simulink model "omav_allocation"  (R2020a)
settings: Solver=VariableStepAuto  StartTime=0.0  StopTime=50  RelTol=1e-3
undefined symbols (not defined in the file): params
libraries: simulink x12
settings Model: Creator=daniel  LastModifiedBy=daniel

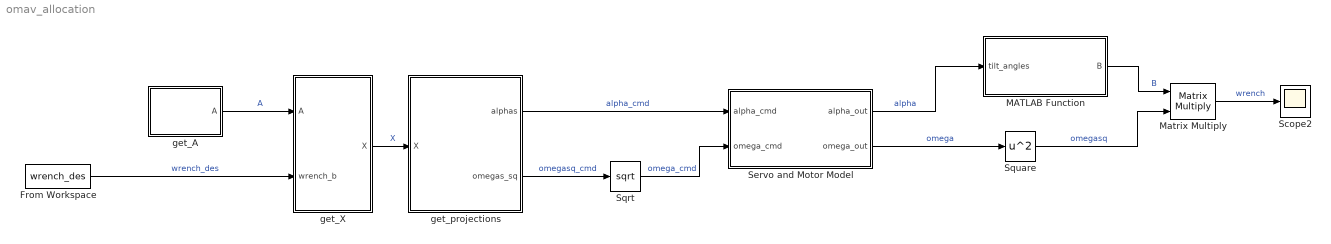
== system omav_allocation ==
  " get_A" : MATLAB Function  TreatAsAtomicUnit=on
  From Workspace : FromWorkspace  VariableName=wrench_des  SampleTime=params.sampling_time
  MATLAB Function : MATLAB Function  TreatAsAtomicUnit=on
  Matrix Multiply : Product  Multiplication=Matrix(*)
  Scope2 : Scope
  Servo and Motor Model : Subsystem
  Sqrt : Sqrt  SaturateOnIntegerOverflow=on
  Square : Math  Operator=square  SaturateOnIntegerOverflow=on
  get_X : MATLAB Function  TreatAsAtomicUnit=on
  get_projections : MATLAB Function  TreatAsAtomicUnit=on
  wires:
  From Workspace/1 -> get_X/2(wrench_b)  "wrench_des"
  " get_A"/1(A) -> get_X/1(A)  "A"
  get_X/1(X) -> get_projections/1(X)  "X"
  get_projections/1(alphas) -> Servo and Motor Model/1(alpha_cmd)  "alpha_cmd"
  MATLAB Function/1(B) -> Matrix Multiply/1  "B"
  get_projections/2(omegas_sq) -> Sqrt/1  "omegasq_cmd"
  Matrix Multiply/1 -> Scope2/1  "wrench"
  Sqrt/1 -> Servo and Motor Model/2(omega_cmd)  "omega_cmd"
  Servo and Motor Model/1(alpha_out) -> MATLAB Function/1(tilt_angles)  "alpha"
  Servo and Motor Model/2(omega_out) -> Square/1  "omega"
  Square/1 -> Matrix Multiply/2  "omegasq"

== system omav_allocation/Servo and Motor Model ==
  alpha_cmd : Inport
  omega_cmd : Inport  Port=2
  all_rotors_subsystem1 : Subsystem
      mask Display: image('images/brushless.JPG'); % Use "Edit Image" on toolstrip to change.
  all_servos_subsystem1 : Subsystem
      mask Display: image('images/servo.jpg'); % Use "Edit Image" on toolstrip to change.
  alpha_out : Outport
  omega_out : Outport  Port=2
  wires:
  alpha_cmd/1 -> all_servos_subsystem1/1(alphas_cmd)  "alpha_cmd"
  all_rotors_subsystem1/1(omegas_out) -> omega_out/1  "omega_out"
  all_servos_subsystem1/1(alphas_out) -> alpha_out/1  "alpha_out"
  omega_cmd/1 -> all_rotors_subsystem1/1(omegas_cmd)  "omega_cmd"

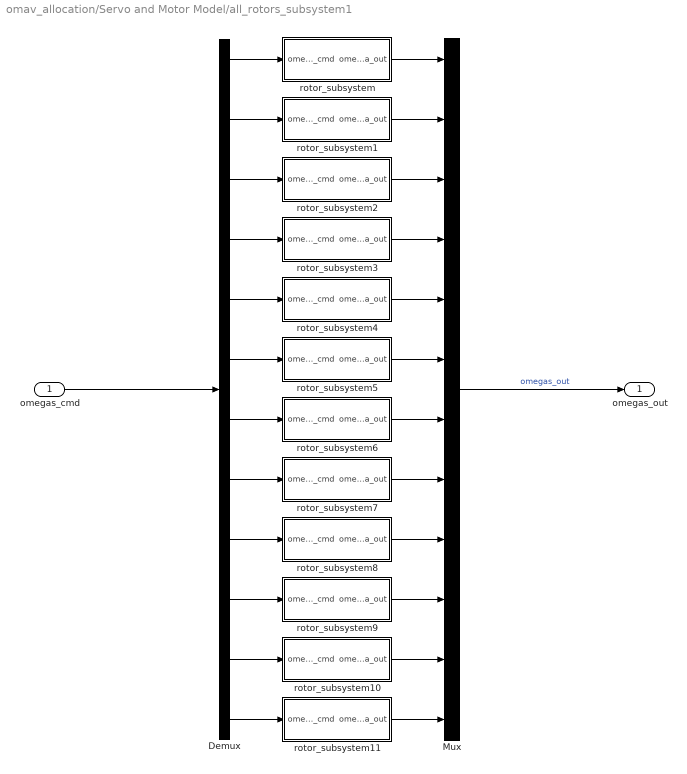
== system omav_allocation/Servo and Motor Model/all_rotors_subsystem1 ==
  omegas_cmd : Inport
  Demux : Demux  Outputs=12
  Mux : Mux  Inputs=12
  rotor_subsystem : Subsystem
  rotor_subsystem1 : Subsystem
  rotor_subsystem10 : Subsystem
  rotor_subsystem11 : Subsystem
  rotor_subsystem2 : Subsystem
  rotor_subsystem3 : Subsystem
  rotor_subsystem4 : Subsystem
  rotor_subsystem5 : Subsystem
  rotor_subsystem6 : Subsystem
  rotor_subsystem7 : Subsystem
  rotor_subsystem8 : Subsystem
  rotor_subsystem9 : Subsystem
  omegas_out : Outport
  wires:
  Demux/3 -> rotor_subsystem2/1(omega_cmd)
  rotor_subsystem10/1(omega_out) -> Mux/11
  rotor_subsystem7/1(omega_out) -> Mux/8
  rotor_subsystem2/1(omega_out) -> Mux/3
  rotor_subsystem1/1(omega_out) -> Mux/2
  Demux/2 -> rotor_subsystem1/1(omega_cmd)
  rotor_subsystem5/1(omega_out) -> Mux/6
  rotor_subsystem4/1(omega_out) -> Mux/5
  Demux/4 -> rotor_subsystem3/1(omega_cmd)
  rotor_subsystem6/1(omega_out) -> Mux/7
  Demux/8 -> rotor_subsystem7/1(omega_cmd)
  rotor_subsystem/1(omega_out) -> Mux/1
  rotor_subsystem3/1(omega_out) -> Mux/4
  rotor_subsystem11/1(omega_out) -> Mux/12
  rotor_subsystem8/1(omega_out) -> Mux/9
  Demux/11 -> rotor_subsystem10/1(omega_cmd)
  rotor_subsystem9/1(omega_out) -> Mux/10
  Demux/1 -> rotor_subsystem/1(omega_cmd)
  omegas_cmd/1 -> Demux/1
  Mux/1 -> omegas_out/1  "omegas_out"
  Demux/12 -> rotor_subsystem11/1(omega_cmd)
  Demux/10 -> rotor_subsystem9/1(omega_cmd)
  Demux/9 -> rotor_subsystem8/1(omega_cmd)
  Demux/7 -> rotor_subsystem6/1(omega_cmd)
  Demux/6 -> rotor_subsystem5/1(omega_cmd)
  Demux/5 -> rotor_subsystem4/1(omega_cmd)

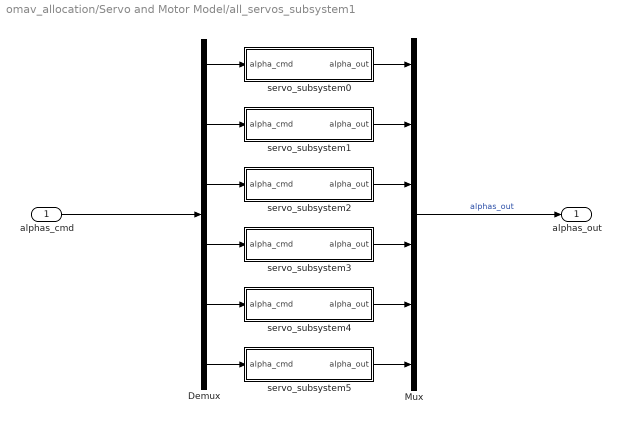
== system omav_allocation/Servo and Motor Model/all_servos_subsystem1 ==
  alphas_cmd : Inport
  Demux : Demux  Outputs=6
  Mux : Mux  Inputs=6
  servo_subsystem0 : Subsystem
  servo_subsystem1 : Subsystem
  servo_subsystem2 : Subsystem
  servo_subsystem3 : Subsystem
  servo_subsystem4 : Subsystem
  servo_subsystem5 : Subsystem
  alphas_out : Outport
  wires:
  alphas_cmd/1 -> Demux/1
  Demux/2 -> servo_subsystem1/1(alpha_cmd)
  servo_subsystem3/1(alpha_out) -> Mux/4
  servo_subsystem1/1(alpha_out) -> Mux/2
  Demux/4 -> servo_subsystem3/1(alpha_cmd)
  servo_subsystem4/1(alpha_out) -> Mux/5
  Demux/5 -> servo_subsystem4/1(alpha_cmd)
  Demux/1 -> servo_subsystem0/1(alpha_cmd)
  servo_subsystem2/1(alpha_out) -> Mux/3
  servo_subsystem5/1(alpha_out) -> Mux/6
  Demux/6 -> servo_subsystem5/1(alpha_cmd)
  Demux/3 -> servo_subsystem2/1(alpha_cmd)
  Mux/1 -> alphas_out/1  "alphas_out"
  servo_subsystem0/1(alpha_out) -> Mux/1

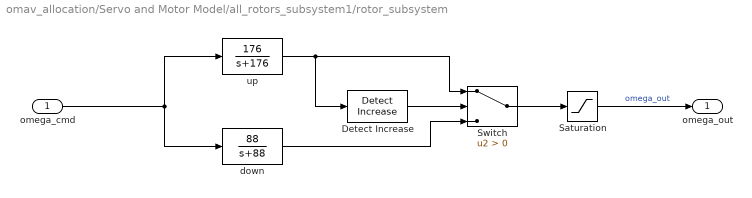
== system omav_allocation/Servo and Motor Model/all_rotors_subsystem1/rotor_subsystem ==
  omega_cmd : Inport
  Detect Increase : simulink/Logic and Bit Operations/Detect Increase  vinit=0.0  OutDataTypeStr=boolean
  Saturation : Saturate  UpperLimit=params.rotor_max  LowerLimit=0
  Switch : Switch  Criteria=u2 > Threshold
  down : TransferFcn  Numerator=[88]  Denominator=[1 88]
  up : TransferFcn  Numerator=[176]  Denominator=[1 176]
  omega_out : Outport
  wires:
  down/1 -> Switch/3
  up/1 -> Detect Increase/1, Switch/1
  omega_cmd/1 -> up/1, down/1
  Switch/1 -> Saturation/1
  Detect Increase/1 -> Switch/2
  Saturation/1 -> omega_out/1  "omega_out"

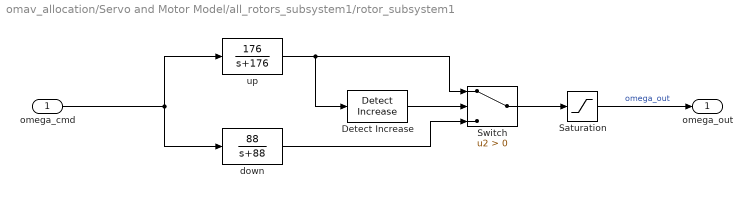
== system omav_allocation/Servo and Motor Model/all_rotors_subsystem1/rotor_subsystem1 ==
  omega_cmd : Inport
  Detect Increase : simulink/Logic and Bit Operations/Detect Increase  vinit=0.0  OutDataTypeStr=boolean
  Saturation : Saturate  UpperLimit=params.rotor_max  LowerLimit=0
  Switch : Switch  Criteria=u2 > Threshold
  down : TransferFcn  Numerator=[88]  Denominator=[1 88]
  up : TransferFcn  Numerator=[176]  Denominator=[1 176]
  omega_out : Outport
  wires:
  Saturation/1 -> omega_out/1  "omega_out"
  Detect Increase/1 -> Switch/2
  Switch/1 -> Saturation/1
  omega_cmd/1 -> down/1, up/1
  up/1 -> Switch/1, Detect Increase/1
  down/1 -> Switch/3

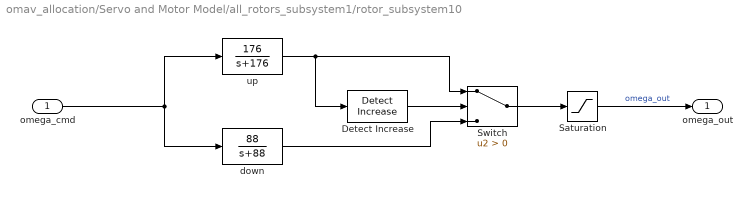
== system omav_allocation/Servo and Motor Model/all_rotors_subsystem1/rotor_subsystem10 ==
  omega_cmd : Inport
  Detect Increase : simulink/Logic and Bit Operations/Detect Increase  vinit=0.0  OutDataTypeStr=boolean
  Saturation : Saturate  UpperLimit=params.rotor_max  LowerLimit=0
  Switch : Switch  Criteria=u2 > Threshold
  down : TransferFcn  Numerator=[88]  Denominator=[1 88]
  up : TransferFcn  Numerator=[176]  Denominator=[1 176]
  omega_out : Outport
  wires:
  down/1 -> Switch/3
  up/1 -> Detect Increase/1, Switch/1
  omega_cmd/1 -> up/1, down/1
  Switch/1 -> Saturation/1
  Detect Increase/1 -> Switch/2
  Saturation/1 -> omega_out/1  "omega_out"

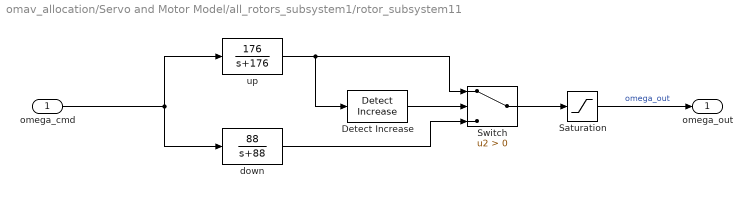
== system omav_allocation/Servo and Motor Model/all_rotors_subsystem1/rotor_subsystem11 ==
  omega_cmd : Inport
  Detect Increase : simulink/Logic and Bit Operations/Detect Increase  vinit=0.0  OutDataTypeStr=boolean
  Saturation : Saturate  UpperLimit=params.rotor_max  LowerLimit=0
  Switch : Switch  Criteria=u2 > Threshold
  down : TransferFcn  Numerator=[88]  Denominator=[1 88]
  up : TransferFcn  Numerator=[176]  Denominator=[1 176]
  omega_out : Outport
  wires:
  Saturation/1 -> omega_out/1  "omega_out"
  Detect Increase/1 -> Switch/2
  Switch/1 -> Saturation/1
  omega_cmd/1 -> down/1, up/1
  up/1 -> Switch/1, Detect Increase/1
  down/1 -> Switch/3

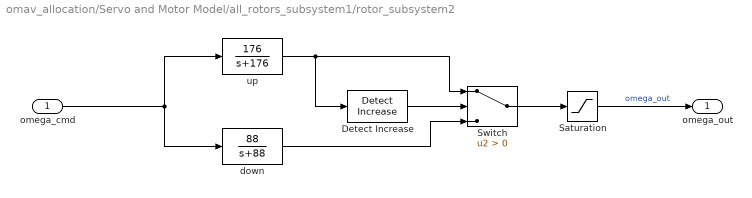
== system omav_allocation/Servo and Motor Model/all_rotors_subsystem1/rotor_subsystem2 ==
  omega_cmd : Inport
  Detect Increase : simulink/Logic and Bit Operations/Detect Increase  vinit=0.0  OutDataTypeStr=boolean
  Saturation : Saturate  UpperLimit=params.rotor_max  LowerLimit=0
  Switch : Switch  Criteria=u2 > Threshold
  down : TransferFcn  Numerator=[88]  Denominator=[1 88]
  up : TransferFcn  Numerator=[176]  Denominator=[1 176]
  omega_out : Outport
  wires:
  down/1 -> Switch/3
  up/1 -> Detect Increase/1, Switch/1
  omega_cmd/1 -> up/1, down/1
  Switch/1 -> Saturation/1
  Detect Increase/1 -> Switch/2
  Saturation/1 -> omega_out/1  "omega_out"

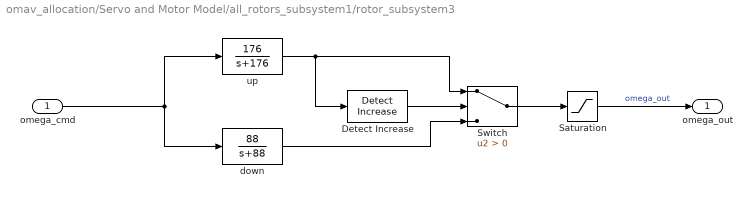
== system omav_allocation/Servo and Motor Model/all_rotors_subsystem1/rotor_subsystem3 ==
  omega_cmd : Inport
  Detect Increase : simulink/Logic and Bit Operations/Detect Increase  vinit=0.0  OutDataTypeStr=boolean
  Saturation : Saturate  UpperLimit=params.rotor_max  LowerLimit=0
  Switch : Switch  Criteria=u2 > Threshold
  down : TransferFcn  Numerator=[88]  Denominator=[1 88]
  up : TransferFcn  Numerator=[176]  Denominator=[1 176]
  omega_out : Outport
  wires:
  Saturation/1 -> omega_out/1  "omega_out"
  Detect Increase/1 -> Switch/2
  Switch/1 -> Saturation/1
  omega_cmd/1 -> down/1, up/1
  up/1 -> Switch/1, Detect Increase/1
  down/1 -> Switch/3

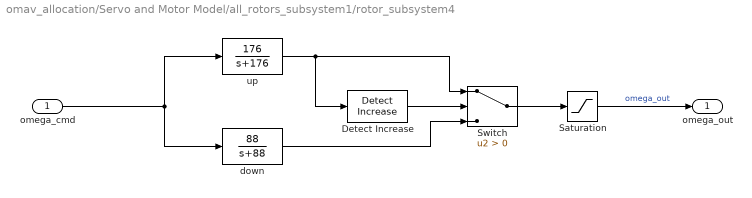
== system omav_allocation/Servo and Motor Model/all_rotors_subsystem1/rotor_subsystem4 ==
  omega_cmd : Inport
  Detect Increase : simulink/Logic and Bit Operations/Detect Increase  vinit=0.0  OutDataTypeStr=boolean
  Saturation : Saturate  UpperLimit=params.rotor_max  LowerLimit=0
  Switch : Switch  Criteria=u2 > Threshold
  down : TransferFcn  Numerator=[88]  Denominator=[1 88]
  up : TransferFcn  Numerator=[176]  Denominator=[1 176]
  omega_out : Outport
  wires:
  down/1 -> Switch/3
  up/1 -> Detect Increase/1, Switch/1
  omega_cmd/1 -> up/1, down/1
  Switch/1 -> Saturation/1
  Detect Increase/1 -> Switch/2
  Saturation/1 -> omega_out/1  "omega_out"

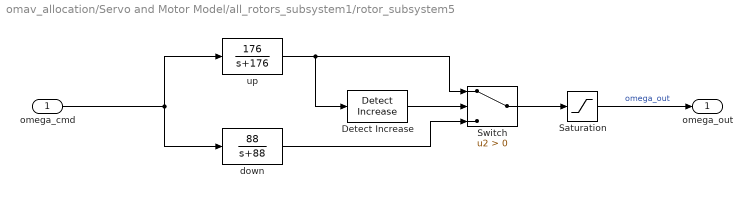
== system omav_allocation/Servo and Motor Model/all_rotors_subsystem1/rotor_subsystem5 ==
  omega_cmd : Inport
  Detect Increase : simulink/Logic and Bit Operations/Detect Increase  vinit=0.0  OutDataTypeStr=boolean
  Saturation : Saturate  UpperLimit=params.rotor_max  LowerLimit=0
  Switch : Switch  Criteria=u2 > Threshold
  down : TransferFcn  Numerator=[88]  Denominator=[1 88]
  up : TransferFcn  Numerator=[176]  Denominator=[1 176]
  omega_out : Outport
  wires:
  Saturation/1 -> omega_out/1  "omega_out"
  Detect Increase/1 -> Switch/2
  Switch/1 -> Saturation/1
  omega_cmd/1 -> down/1, up/1
  up/1 -> Switch/1, Detect Increase/1
  down/1 -> Switch/3

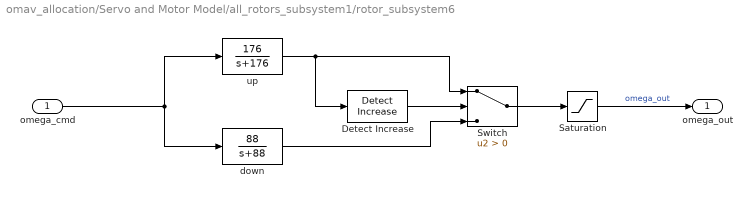
== system omav_allocation/Servo and Motor Model/all_rotors_subsystem1/rotor_subsystem6 ==
  omega_cmd : Inport
  Detect Increase : simulink/Logic and Bit Operations/Detect Increase  vinit=0.0  OutDataTypeStr=boolean
  Saturation : Saturate  UpperLimit=params.rotor_max  LowerLimit=0
  Switch : Switch  Criteria=u2 > Threshold
  down : TransferFcn  Numerator=[88]  Denominator=[1 88]
  up : TransferFcn  Numerator=[176]  Denominator=[1 176]
  omega_out : Outport
  wires:
  down/1 -> Switch/3
  up/1 -> Detect Increase/1, Switch/1
  omega_cmd/1 -> up/1, down/1
  Switch/1 -> Saturation/1
  Detect Increase/1 -> Switch/2
  Saturation/1 -> omega_out/1  "omega_out"

== system omav_allocation/Servo and Motor Model/all_rotors_subsystem1/rotor_subsystem7 ==
  omega_cmd : Inport
  Detect Increase : simulink/Logic and Bit Operations/Detect Increase  vinit=0.0  OutDataTypeStr=boolean
  Saturation : Saturate  UpperLimit=params.rotor_max  LowerLimit=0
  Switch : Switch  Criteria=u2 > Threshold
  down : TransferFcn  Numerator=[88]  Denominator=[1 88]
  up : TransferFcn  Numerator=[176]  Denominator=[1 176]
  omega_out : Outport
  wires:
  Saturation/1 -> omega_out/1  "omega_out"
  Detect Increase/1 -> Switch/2
  Switch/1 -> Saturation/1
  omega_cmd/1 -> down/1, up/1
  up/1 -> Switch/1, Detect Increase/1
  down/1 -> Switch/3

== system omav_allocation/Servo and Motor Model/all_rotors_subsystem1/rotor_subsystem8 ==
  omega_cmd : Inport
  Detect Increase : simulink/Logic and Bit Operations/Detect Increase  vinit=0.0  OutDataTypeStr=boolean
  Saturation : Saturate  UpperLimit=params.rotor_max  LowerLimit=0
  Switch : Switch  Criteria=u2 > Threshold
  down : TransferFcn  Numerator=[88]  Denominator=[1 88]
  up : TransferFcn  Numerator=[176]  Denominator=[1 176]
  omega_out : Outport
  wires:
  down/1 -> Switch/3
  up/1 -> Detect Increase/1, Switch/1
  omega_cmd/1 -> up/1, down/1
  Switch/1 -> Saturation/1
  Detect Increase/1 -> Switch/2
  Saturation/1 -> omega_out/1  "omega_out"

== system omav_allocation/Servo and Motor Model/all_rotors_subsystem1/rotor_subsystem9 ==
  omega_cmd : Inport
  Detect Increase : simulink/Logic and Bit Operations/Detect Increase  vinit=0.0  OutDataTypeStr=boolean
  Saturation : Saturate  UpperLimit=params.rotor_max  LowerLimit=0
  Switch : Switch  Criteria=u2 > Threshold
  down : TransferFcn  Numerator=[88]  Denominator=[1 88]
  up : TransferFcn  Numerator=[176]  Denominator=[1 176]
  omega_out : Outport
  wires:
  Saturation/1 -> omega_out/1  "omega_out"
  Detect Increase/1 -> Switch/2
  Switch/1 -> Saturation/1
  omega_cmd/1 -> down/1, up/1
  up/1 -> Switch/1, Detect Increase/1
  down/1 -> Switch/3

== system omav_allocation/Servo and Motor Model/all_servos_subsystem1/servo_subsystem0 ==
  alpha_cmd : Inport
  Servo Transfer Function : TransferFcn  Numerator=[256]  Denominator=[1 22.4 256]
  alpha_out : Outport
  wires:
  alpha_cmd/1 -> Servo Transfer Function/1
  Servo Transfer Function/1 -> alpha_out/1  "alpha_out"

== system omav_allocation/Servo and Motor Model/all_servos_subsystem1/servo_subsystem1 ==
  alpha_cmd : Inport
  Servo Transfer Function : TransferFcn  Numerator=[256]  Denominator=[1 22.4 256]
  alpha_out : Outport
  wires:
  Servo Transfer Function/1 -> alpha_out/1  "alpha_out"
  alpha_cmd/1 -> Servo Transfer Function/1

== system omav_allocation/Servo and Motor Model/all_servos_subsystem1/servo_subsystem2 ==
  alpha_cmd : Inport
  Servo Transfer Function : TransferFcn  Numerator=[256]  Denominator=[1 22.4 256]
  alpha_out : Outport
  wires:
  alpha_cmd/1 -> Servo Transfer Function/1
  Servo Transfer Function/1 -> alpha_out/1  "alpha_out"

== system omav_allocation/Servo and Motor Model/all_servos_subsystem1/servo_subsystem3 ==
  alpha_cmd : Inport
  Servo Transfer Function : TransferFcn  Numerator=[256]  Denominator=[1 22.4 256]
  alpha_out : Outport
  wires:
  Servo Transfer Function/1 -> alpha_out/1  "alpha_out"
  alpha_cmd/1 -> Servo Transfer Function/1

== system omav_allocation/Servo and Motor Model/all_servos_subsystem1/servo_subsystem4 ==
  alpha_cmd : Inport
  Servo Transfer Function : TransferFcn  Numerator=[256]  Denominator=[1 22.4 256]
  alpha_out : Outport
  wires:
  alpha_cmd/1 -> Servo Transfer Function/1
  Servo Transfer Function/1 -> alpha_out/1  "alpha_out"

== system omav_allocation/Servo and Motor Model/all_servos_subsystem1/servo_subsystem5 ==
  alpha_cmd : Inport
  Servo Transfer Function : TransferFcn  Numerator=[256]  Denominator=[1 22.4 256]
  alpha_out : Outport
  wires:
  Servo Transfer Function/1 -> alpha_out/1  "alpha_out"
  alpha_cmd/1 -> Servo Transfer Function/1

== matlab function omav_allocation/get_X ==
  data: A input; X output; wrench_b input
function X = get_X(A,wrench_b)
%GET_X Summary of this function goes here
%   Detailed explanation goes here

X = pinv(A)*wrench_b;
end

== matlab function omav_allocation/get_projections ==
  data: X input; alphas output; omegas_sq output
function [alphas, omegas_sq] = get_projections(X)
%GET_PROJECTIONS Summary of this function goes here
%   Detailed explanation goes here


%get the angles
alphas = zeros(6,1);
for i = 1:6
    %get to entry which corresponds to arm
    j = 4*i - 3;
    alphas(i) = atan2(X(j)+X(j+2),X(j+1)+X(j+3));
end

omegas_sq = zeros(12,1);
for i = 1:6
    %get to entry which corresponds to arm
    j = 4*i - 3;
    
    omegas_sq(2*i-1) = X(j)*sin(alphas(i)) + X(j+1)*cos(alphas(i));
    omegas_sq(2*i)   = X(j+2)*sin(alphas(i)) + X(j+3)*cos(alphas(i));
end

%set to zero if smaller than zero
for i = 1:12
    if omegas_sq(i) < 0
        omegas_sq(i) = 0;
    end
end

== matlab function omav_allocation/MATLAB Function ==
  data: tilt_angles input; B output
function B = get_B(tilt_angles)
%tilt_angles [6x1]
%[F, tau] = B * [omega²]

params = parameters();

rotor_force_constant = params.rotor_force_constant;
rotor_moment_constant = params.rotor_moment_constant;
arm_length = params.arm_length;

arm_angles = params.arm_angles;
spin = params.spin;

B = zeros(6,12);


j = 0;

%repeat every tilt angle
rep_tilt_angles = repelem(tilt_angles,2);
%iterating through every rotor
for i = 1:12
  
    tilt_angle = rep_tilt_angles(i);
    
    
    B(1,i) = -sin(arm_angles(i))*sin(tilt_angle);
    B(2,i) = cos(arm_angles(i))*sin(tilt_angle);
    B(3,i) = -cos(tilt_angle);
    B(4,i) = -(rotor_moment_constant*spin(i)*sin(tilt_angle) + cos(tilt_angle)*arm_length)*sin(arm_angles(i));
    B(5,i) =  (rotor_moment_constant*spin(i)*sin(tilt_angle) + cos(tilt_angle)*arm_length)*cos(arm_angles(i));
    B(6,i) = -rotor_moment_constant*spin(i)*cos(tilt_angle) + sin(tilt_angle)*arm_length;
end

B = B*rotor_force_constant;

== matlab function omav_allocation/ get_A ==
  data: A output
function A = get_A()
%[F, tau] = A * [sin(alpha)*omega², cos(alpha)*omega²]

params = parameters();

rotor_force_constant = params.rotor_force_constant;
rotor_moment_constant = params.rotor_moment_constant;
arm_length = params.arm_length;

arm_angles = params.arm_angles;
spin = params.spin;

%implementing pre-calculated matrix
%zero entries are commented out
A = zeros(6,24);

%iterating through every rotor
for i = 1:12
    A(1,2*i-1) = -sin(arm_angles(i));
    %A(1,2*i) = 0;
    
    A(2,2*i-1) = cos(arm_angles(i));
    %A(2,2*i) = 0;
    
    %A(3,2*i-1) = 0;
    A(3,2*i) = -1;
    
    A(4,2*i-1) = -rotor_moment_constant*spin(i)*sin(arm_angles(i));
    A(4,2*i) = -sin(arm_angles(i))*arm_length;
    
    A(5,2*i-1) = rotor_moment_constant*spin(i)*cos(arm_angles(i));
    A(5,2*i) = cos(arm_angles(i))*arm_length;
    
    A(6,2*i-1) = arm_length;
    A(6,2*i) = -rotor_moment_constant*spin(i);
end

%multiplying with rotor force constant
A = A*rotor_force_constant;
